simulink model "irb1600"  (R2022b)
settings: Solver=VariableStepAuto  StartTime=0.0  StopTime=5  RelTol=1e-3
undefined symbols (not defined in the file or in its folder): inputvar
libraries: robotmaniplib x2, slpidlib x1
settings Model: Creator=paulcrann  LastModifiedBy=paulcrann

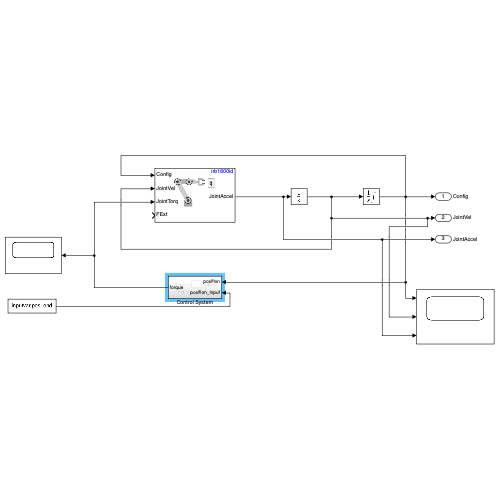
[thumbnail: Simulink's stored preview of the top-level diagram]
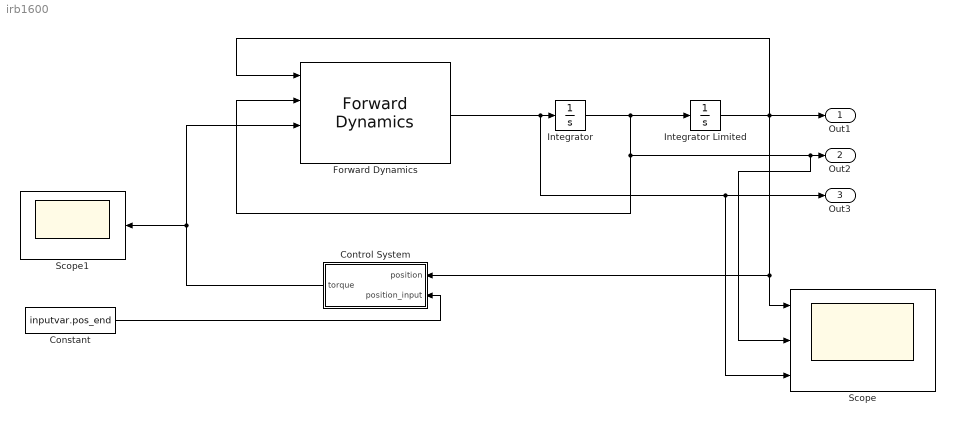
== system irb1600 ==
  Constant : Constant  Value=inputvar.pos_end
  Control System : Subsystem
  Forward Dynamics : robotmaniplib/Forward Dynamics  RigidBodyTree=irb1600id  SimulateUsing=Interpreted execution
  Integrator : Integrator  InitialCondition=inputvar.vel_0
  Integrator Limited : Integrator  InitialCondition=inputvar.pos_0  LimitOutput=on  UpperSaturationLimit=pi  LowerSaturationLimit=-pi
  Scope : Scope  NumInputPorts=3
  Scope1 : Scope
  Out1 : Outport  SignalName=Config  OutDataTypeStr=double
  Out2 : Outport  Port=2  SignalName=JointVel
  Out3 : Outport  Port=3  SignalName=JointAccel
  wires:
  Forward Dynamics/1 -> Out3/1, Scope/3, Integrator/1
  Integrator/1 -> Forward Dynamics/2, Scope/2, Out2/1, Integrator Limited/1
  Integrator Limited/1 -> Scope/1, Control System/1(position), Forward Dynamics/1, Out1/1
  Control System/1(torque) -> Scope1/1, Forward Dynamics/3
  Constant/1 -> Control System/2(position_input)

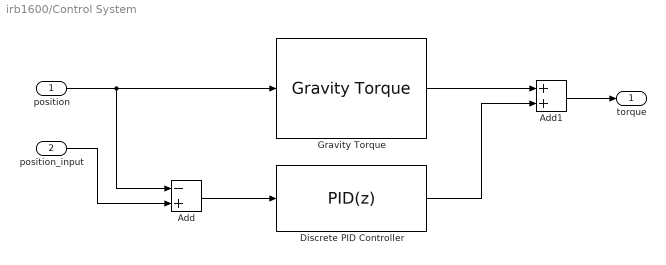
== system irb1600/Control System ==
  position : Inport
  position_input : Inport  Port=2
  Add : Sum  Inputs=-+
  Add1 : Sum
  Discrete PID Controller : slpidlib/PID Controller  Controller=PID  Form=Parallel  TimeDomain=Discrete-time  UseExternalTs=off  SampleTime=-1  IntegratorMethod=Forward Euler  FilterMethod=Forward Euler  ControllerParametersSource=internal  P=inputvar.PID.P  I=inputvar.PID.I  UseKiTs=on  D=inputvar.PID.D  N=5  UseFilter=on  TunerSelectOption=Transfer Function Based (PID Tuner App)  InitialConditionSource=internal  InitialConditionForIntegrator=0  InitialConditionForFilter=0  DifferentiatorICPrevScaledInput=0  ExternalReset=none  TrackingMode=off  Kt=1  LimitOutput=off  SatLimitsSource=internal  UpperSaturationLimit=inf  LowerSaturationLimit=-inf  LinearizeAsGain=off  AntiWindupMode=none  Kb=1  LimitIntegrator=off  UpperIntegratorSaturationLimit=inf  LowerIntegratorSaturationLimit=-inf  POutMin=[]  POutMax=[]  IOutMin=[]  IOutMax=[]  DOutMin=[]  DOutMax=[]  NOutMin=[]  NOutMax=[]  SumOutMin=[]  SumOutMax=[]  SaturationOutMin=[]  SaturationOutMax=[]  PParamMin=[]  PParamMax=[]  IParamMin=[]  IParamMax=[]  DParamMin=[]  DParamMax=[]  NParamMin=[]  NParamMax=[]  KbParamMin=[]  KbParamMax=[]  KtParamMin=[]  KtParamMax=[]  KbOutMin=[]  KbOutMax=[]  KtOutMin=[]  KtOutMax=[]  IntegratorOutMin=[]  IntegratorOutMax=[]  FilterOutMin=[]  FilterOutMax=[]  SumI1OutMin=[]  SumI1OutMax=[]  SumI2OutMin=[]  SumI2OutMax=[]  SumI3OutMin=[]  SumI3OutMax=[]  SumI4OutMin=[]  SumI4OutMax=[]  SumDOutMin=[]  SumDOutMax=[]  DifferentiatorOutMin=[]  DifferentiatorOutMax=[]  FilterDiffOutCoefMin=[]  FilterDiffOutCoefMax=[]  ReciprocalOutMin=[]  ReciprocalOutMax=[]  SumDenOutMin=[]  SumDenOutMax=[]  SumNumOutMin=[]  SumNumOutMax=[]  DivideOutMin=[]  DivideOutMax=[]  UdiffTsProdOutMin=[]  UdiffTsProdOutMax=[]  NTsProdOutMin=[]  NTsProdOutMax=[]  UintegralTsProdOutMin=[]  UintegralTsProdOutMax=[]  UngainTsProdOutMin=[]  UngainTsProdOutMax=[]  ClampingZeroOutDataTypeStr=Inherit: Inherit via back propagation  ClampingZeroOutMin=[]  ClampingZeroOutMax=[]  FilterDenConstantOutDataTypeStr=Inherit: Inherit via back propagation  FilterDenConstantOutMin=[]  FilterDenConstantOutMax=[]  PCopyOutDataTypeStr=Inherit: Inherit via back propagation  PCopyOutMin=[]  PCopyOutMax=[]  NCopyOutDataTypeStr=Inherit: Inherit via back propagation  NCopyOutMin=[]  NCopyOutMax=[]  IntegratorContinuousStateAttributes=''  IntegratorStateMustResolveToSignalObject=off  IntegratorRTWStateStorageClass=Auto  FilterContinuousStateAttributes=''  FilterStateMustResolveToSignalObject=off  FilterRTWStateStorageClass=Auto  ParallelPVariant=InternalParameters  IdealPVariant=Disabled  IVariant=InternalParameters  DVariant=InternalParameters  IntegratorVariant=Discrete  SatVariant=Disabled  AWVariant=Passthrough  PCopyVariant=Disabled  TRVariant=Disabled  FdbkBlocksVariant=Forward  IdealPFdbkVariant=Disabled  SatFdbkVariant=Disabled  DerivativeFilterVariant=ForwardEulerFilter  NVariant=InternalParameters  NCopyVariant=Disabled  FilterICVariant=InternalICsFilter  IntegratorICVariant=InternalICs  ExternalResetVariant=Disabled  TRSumVariant=Passthrough  SumFdbkVariant=Disabled  SumVariant=Sum_PID  TsampFilterVariant=InternalTs  TsampNgainVariant=Passthrough  TsampIntegralVariant=Passthrough  ExternalSaturationOutDataTypeStr=Inherit: Same as second input
      settings: LibrarySourceBlock=simulink/Discrete/Discrete PID Controller
  Gravity Torque : robotmaniplib/Gravity Torque  RigidBodyTree=irb1600id  SimulateUsing=Interpreted execution
  torque : Outport
  wires:
  position/1 -> Gravity Torque/1, Add/1
  position_input/1 -> Add/2
  Add/1 -> Discrete PID Controller/1
  Gravity Torque/1 -> Add1/1
  Discrete PID Controller/1 -> Add1/2
  Add1/1 -> torque/1
